simulink model "Project6"  (R2014a)
settings: Solver=ode45  StartTime=0.0  StopTime=310  RelTol=1e-3
undefined symbols (not defined in the file or in its folder): AXI4, Lite
libraries: xbsIndex_r4 x267
(part 1 of 2)
settings Model: Creator=Uday Kiran  LastModifiedBy=uk3
settings DebuggingCC: SolverPrmCheckMsg=none

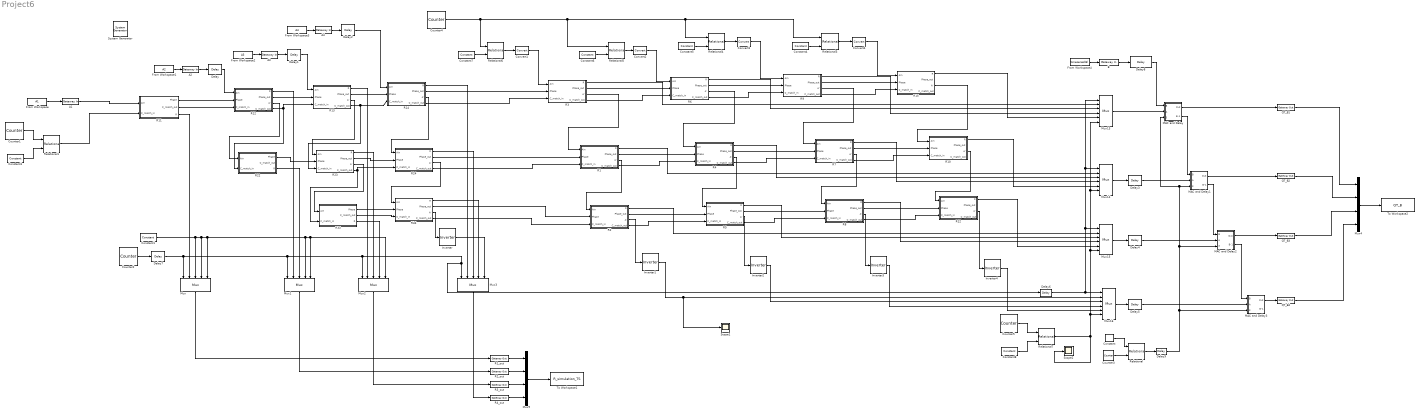
== system Project6 ==
  " System Generator" : xbsIndex_r4/ System Generator  Tag=genX  xilinxfamily=zynq  part=xc7z020  speed=-1  package=clg484  synthesis_tool=Vivado  clock_wrapper=Clock Enables  directory=./netlist  proj_type=Vivado  Synth_file=Vivado Synthesis Defaults  Impl_file=Vivado Implementation Defaults  testbench=off  simulink_period=1  sysclk_period=10  dcm_input_clock_period=10  incr_netlist=off  trim_vbits=Everywhere in SubSystem  dbl_ovrd=According to Block Masks  core_generation=According to Block Masks  run_coregen=off  deprecated_control=off  eval_field=0  block_type=sysgen
  A{1..4} (4 alike) : xbsIndex_r4/Gateway In  gui_display_data_type=Fixed-point  arith_type="Signed  (2's comp)"  n_bits=16  bin_pt=14  preci_type=Single  exp_width=8  frac_width=24  quantization="Round  (unbiased: +/- Inf)"  overflow=Saturate  period=1  UseAsADC=off  ADCChannel='1'  interface=AXI4-Lite  automatic_assignment=on  address_offset=hex2dec('00')  intf_description=''  timing_constraint=None  locs_specified=off  LOCs={}  io_standard={}  inherit_from_input=off  hdl_port=on  dbl_ovrd=off  block_type=gatewayin
      settings: block_version=VER_STRING_GOES_HERE
  B : xbsIndex_r4/Gateway In  gui_display_data_type=Fixed-point  arith_type="Signed  (2's comp)"  n_bits=16  bin_pt=14  preci_type=Single  exp_width=8  frac_width=24  quantization="Round  (unbiased: +/- Inf)"  overflow=Saturate  period=1  UseAsADC=off  ADCChannel='1'  interface=AXI4-Lite  automatic_assignment=on  address_offset=hex2dec('00')  intf_description=''  timing_constraint=None  locs_specified=off  LOCs={}  io_standard={}  inherit_from_input=off  hdl_port=on  dbl_ovrd=off  block_type=gatewayin
  Constant : xbsIndex_r4/Constant  const=8  gui_display_data_type=Fixed-point  arith_type=Signed (2's comp)  n_bits=16  bin_pt=0  preci_type=Single  exp_width=8  frac_width=24  explicit_period=on  period=1  equ=P=C  opselect=C  inp2=PCIN>>17  opr=+  inp1=P  carry=CIN  dbl_ovrd=off  block_type=constant
  Constant1 : xbsIndex_r4/Constant  const=0  gui_display_data_type=Fixed-point  arith_type=Signed (2's comp)  n_bits=16  bin_pt=14  preci_type=Single  exp_width=8  frac_width=24  explicit_period=off  period=1  equ=P=C  opselect=C  inp2=PCIN>>17  opr=+  inp1=P  carry=CIN  dbl_ovrd=off  block_type=constant
  Constant3 : xbsIndex_r4/Constant  const=0  gui_display_data_type=Fixed-point  arith_type=Signed (2's comp)  n_bits=8  bin_pt=0  preci_type=Single  exp_width=8  frac_width=24  explicit_period=off  period=1  equ=P=C  opselect=C  inp2=PCIN>>17  opr=+  inp1=P  carry=CIN  dbl_ovrd=off  block_type=constant
  Constant4 : xbsIndex_r4/Constant  const=7  gui_display_data_type=Fixed-point  arith_type=Signed (2's comp)  n_bits=10  bin_pt=0  preci_type=Single  exp_width=8  frac_width=24  explicit_period=off  period=1  equ=P=C  opselect=C  inp2=PCIN>>17  opr=+  inp1=P  carry=CIN  dbl_ovrd=off  block_type=constant
  Constant5 : xbsIndex_r4/Constant  const=54  gui_display_data_type=Fixed-point  arith_type=Signed (2's comp)  n_bits=10  bin_pt=0  preci_type=Single  exp_width=8  frac_width=24  explicit_period=off  period=1  equ=P=C  opselect=C  inp2=PCIN>>17  opr=+  inp1=P  carry=CIN  dbl_ovrd=off  block_type=constant
  Constant6 : xbsIndex_r4/Constant  const=101  gui_display_data_type=Fixed-point  arith_type=Signed (2's comp)  n_bits=10  bin_pt=0  preci_type=Single  exp_width=8  frac_width=24  explicit_period=off  period=1  equ=P=C  opselect=C  inp2=PCIN>>17  opr=+  inp1=P  carry=CIN  dbl_ovrd=off  block_type=constant
  Constant7 : xbsIndex_r4/Constant  const=148  gui_display_data_type=Fixed-point  arith_type=Signed (2's comp)  n_bits=10  bin_pt=0  preci_type=Single  exp_width=8  frac_width=24  explicit_period=off  period=1  equ=P=C  opselect=C  inp2=PCIN>>17  opr=+  inp1=P  carry=CIN  dbl_ovrd=off  block_type=constant
  Constant8 : xbsIndex_r4/Constant  const=296  gui_display_data_type=Fixed-point  arith_type=Signed (2's comp)  n_bits=10  bin_pt=0  preci_type=Single  exp_width=8  frac_width=24  explicit_period=off  period=1  equ=P=C  opselect=C  inp2=PCIN>>17  opr=+  inp1=P  carry=CIN  dbl_ovrd=off  block_type=constant
  Convert{1..4} (4 alike) : xbsIndex_r4/Convert  gui_display_data_type=Fixed-point  arith_type="Signed  (2's comp)"  n_bits=16  bin_pt=14  float_type=Single  exp_bits=8  fraction_bits=24  quantization=Truncate  overflow=Wrap  en=off  latency=0  pipeline=on  dbl_ovrd=off  block_type=convert
  Counter1 : xbsIndex_r4/Counter  cnt_type=Count Limited  cnt_to=47  operation=Up  start_count=0  cnt_by_val=1  arith_type="Signed  (2's comp)"  n_bits=8  bin_pt=0  load_pin=off  rst=off  en=off  explicit_period=on  period=1  use_behavioral_HDL=off  implementation=Fabric  dbl_ovrd=off  block_type=counter
  Counter2 : xbsIndex_r4/Counter  cnt_type=Count Limited  cnt_to=3  operation=Up  start_count=0  cnt_by_val=1  arith_type=Unsigned  n_bits=2  bin_pt=0  load_pin=off  rst=off  en=off  explicit_period=on  period=1  use_behavioral_HDL=off  implementation=Fabric  dbl_ovrd=off  block_type=counter
  Counter3 : xbsIndex_r4/Counter  cnt_type=Count Limited  cnt_to=8  operation=Up  start_count=1  cnt_by_val=1  arith_type=Unsigned  n_bits=5  bin_pt=0  load_pin=off  rst=off  en=off  explicit_period=on  period=1  use_behavioral_HDL=off  implementation=Fabric  dbl_ovrd=off  block_type=counter
  Counter4 : xbsIndex_r4/Counter  cnt_type=Count Limited  cnt_to=193  operation=Up  start_count=0  cnt_by_val=1  arith_type="Signed  (2's comp)"  n_bits=10  bin_pt=0  load_pin=off  rst=off  en=off  explicit_period=on  period=1  use_behavioral_HDL=off  implementation=Fabric  dbl_ovrd=off  block_type=counter
  Counter5 : xbsIndex_r4/Counter  cnt_type=Count Limited  cnt_to=300  operation=Up  start_count=1  cnt_by_val=1  arith_type="Signed  (2's comp)"  n_bits=10  bin_pt=0  load_pin=off  rst=off  en=off  explicit_period=on  period=1  use_behavioral_HDL=off  implementation=Fabric  dbl_ovrd=off  block_type=counter
  Delay : xbsIndex_r4/Delay  rst=off  infoeditControl=Selection of Reset will increase slice count due to use of real FFs and instead of SRLs  en=off  latency=1  reg_retiming=off  dbl_ovrd=off  block_type=delay
  Delay1 : xbsIndex_r4/Delay  rst=off  infoeditControl=Selection of Reset will increase slice count due to use of real FFs and instead of SRLs  en=off  latency=2  reg_retiming=off  dbl_ovrd=off  block_type=delay
  Delay2 : xbsIndex_r4/Delay  rst=off  infoeditControl=Selection of Reset will increase slice count due to use of real FFs and instead of SRLs  en=off  latency=3  reg_retiming=off  dbl_ovrd=off  block_type=delay
  Delay3 : xbsIndex_r4/Delay  rst=off  infoeditControl=Selection of Reset will increase slice count due to use of real FFs and instead of SRLs  en=off  latency=1  reg_retiming=off  dbl_ovrd=off  block_type=delay
  Delay4 : xbsIndex_r4/Delay  rst=off  infoeditControl=Selection of Reset will increase slice count due to use of real FFs and instead of SRLs  en=off  latency=2  reg_retiming=off  dbl_ovrd=off  block_type=delay
  Delay5 : xbsIndex_r4/Delay  rst=off  infoeditControl=Selection of Reset will increase slice count due to use of real FFs and instead of SRLs  en=off  latency=3  reg_retiming=off  dbl_ovrd=off  block_type=delay
  Delay6 : xbsIndex_r4/Delay  rst=off  infoeditControl=Selection of Reset will increase slice count due to use of real FFs and instead of SRLs  en=off  latency=3  reg_retiming=off  dbl_ovrd=off  block_type=delay
  Delay7 : xbsIndex_r4/Delay  rst=off  infoeditControl=Selection of Reset will increase slice count due to use of real FFs and instead of SRLs  en=off  latency=1  reg_retiming=off  dbl_ovrd=off  block_type=delay
  Delay8 : xbsIndex_r4/Delay  rst=off  infoeditControl=Selection of Reset will increase slice count due to use of real FFs and instead of SRLs  en=off  latency=297  reg_retiming=off  dbl_ovrd=off  block_type=delay
  Delay9 : xbsIndex_r4/Delay  rst=off  infoeditControl=Selection of Reset will increase slice count due to use of real FFs and instead of SRLs  en=off  latency=4  reg_retiming=off  dbl_ovrd=off  block_type=delay
  From Workspace : FromWorkspace  VariableName=A1  SampleTime=0  OutputAfterFinalValue=Setting to zero
  From Workspace1 : FromWorkspace  VariableName=A2  SampleTime=0  OutputAfterFinalValue=Setting to zero
  From Workspace2 : FromWorkspace  VariableName=A3  SampleTime=0  OutputAfterFinalValue=Setting to zero
  From Workspace3 : FromWorkspace  VariableName=A4  SampleTime=0  OutputAfterFinalValue=Setting to zero
  From Workspace4 : FromWorkspace  VariableName=timeseries(B)  SampleTime=0  OutputAfterFinalValue=Setting to zero
  Inverter{,1..4} (5 alike) : xbsIndex_r4/Inverter  en=off  latency=0  dbl_ovrd=off  block_type=inv
  MAC and Delay : Subsystem
  MAC and Delay1 : Subsystem
  MAC and Delay2 : Subsystem
  MAC and Delay3 : Subsystem
  Mux{,1..3} (4 alike) : xbsIndex_r4/Mux  inputs=4  en=off  latency=0  precision=Full  arith_type=Unsigned  n_bits=16  bin_pt=14  quantization=Truncate  overflow=Wrap  dbl_ovrd=off  block_type=mux
  Mux{13..16} (4 alike) : xbsIndex_r4/Mux  inputs=4  en=on  latency=1  precision=User Defined  arith_type="Signed  (2's comp)"  n_bits=16  bin_pt=14  quantization=Truncate  overflow=Wrap  dbl_ovrd=off  block_type=mux
  Mux4 : Mux
  Mux9 : Mux
  QT_B{1..4} (4 alike) : xbsIndex_r4/Gateway Out  inherit_from_input=off  hdl_port=on  rows=1  columns=1  UseAsDAC=off  DACChannel='1'  interface=AXI4-Lite  automatic_assignment=on  address_offset=hex2dec('00')  intf_description=''  timing_constraint=None  locs_specified=off  LOCs={}  io_standard={}  block_type=gatewayout
  R1 : Subsystem
  R10 : Subsystem
  R11 : Subsystem
  R12 : Subsystem
  "R12 " : Subsystem
  R13 : Subsystem
  R14 : Subsystem
  R15 : Subsystem
  R1_out : xbsIndex_r4/Gateway Out  inherit_from_input=off  hdl_port=on  rows=1  columns=1  UseAsDAC=off  DACChannel='1'  interface=AXI4-Lite  automatic_assignment=on  address_offset=hex2dec('00')  intf_description=''  timing_constraint=None  locs_specified=off  LOCs={}  io_standard={}  block_type=gatewayout
  R2 : Subsystem
  R22 : Subsystem
  R23 : Subsystem
  R24 : Subsystem
  R2_out : xbsIndex_r4/Gateway Out  inherit_from_input=off  hdl_port=on  rows=1  columns=1  UseAsDAC=off  DACChannel='1'  interface=AXI4-Lite  automatic_assignment=on  address_offset=hex2dec('00')  intf_description=''  timing_constraint=None  locs_specified=off  LOCs={}  io_standard={}  block_type=gatewayout
  R3 : Subsystem
  R33 : Subsystem
  R34 : Subsystem
  R3_out : xbsIndex_r4/Gateway Out  inherit_from_input=off  hdl_port=on  rows=1  columns=1  UseAsDAC=off  DACChannel='1'  interface=AXI4-Lite  automatic_assignment=on  address_offset=hex2dec('00')  intf_description=''  timing_constraint=None  locs_specified=off  LOCs={}  io_standard={}  block_type=gatewayout
  R4 : Subsystem
  R4_out : xbsIndex_r4/Gateway Out  inherit_from_input=off  hdl_port=on  rows=1  columns=1  UseAsDAC=off  DACChannel='1'  interface=AXI4-Lite  automatic_assignment=on  address_offset=hex2dec('00')  intf_description=''  timing_constraint=None  locs_specified=off  LOCs={}  io_standard={}  block_type=gatewayout
  R5 : Subsystem
  R6 : Subsystem
  R7 : Subsystem
  R8 : Subsystem
  R9 : Subsystem
  Relational{,1,3..6} (6 alike) : xbsIndex_r4/Relational  mode=a=b  op_type=Bool  en=off  latency=0  dbl_ovrd=off  block_type=relational
  Relational7 : xbsIndex_r4/Relational  mode=a>b  op_type=Bool  en=off  latency=0  dbl_ovrd=off  block_type=relational
  Scope1 : Scope
  Scope2 : Scope
  To Workspace1 : ToWorkspace  VariableName=R_simulation_TS  SaveFormat=Timeseries  SampleTime=-1
      settings: MaxDataPoints=8
  To Workspace2 : ToWorkspace  VariableName=QT_B  SaveFormat=Timeseries  SampleTime=-1
  wires:
  From Workspace/1 -> A1/1
  From Workspace1/1 -> A2/1
  A1/1 -> R11/1(Ain)
  A2/1 -> Delay/1
  R11/1(Phase) -> "R12 "/2(Phase)
  R11/2(C_match_out) -> "R12 "/3(C_match_in)
  Counter1/1 -> Relational1/1
  Constant3/1 -> Relational1/2
  Relational1/1 -> R11/2("C_match_in ")
  "R12 "/3(A') -> R22/1(Ain)
  "R12 "/4(C_match_out) -> R22/2("C_match_in "), R13/3(C_match_in)
  Delay/1 -> "R12 "/1(Ain)
  "R12 "/2(Phase_out) -> R13/2(Phase)
  R13/2(Phase_out) -> R14/2(Phase)
  R13/3(A') -> R23/1(Ain)
  R23/2(Phase_out) -> R24/2(Phase)
  R14/3(A') -> R24/1(Ain)
  R23/3(A') -> R33/1(Ain)
  R23/4(C_match_out) -> R33/2("C_match_in "), R24/3(C_match_in)
  R33/1(Phase) -> R34/2(Phase)
  R24/3(A') -> R34/1(Ain)
  From Workspace2/1 -> A3/1
  A3/1 -> Delay1/1
  Delay1/1 -> R13/1(Ain)
  From Workspace3/1 -> A4/1
  A4/1 -> Delay2/1
  Delay2/1 -> R14/1(Ain)
  "R12 "/1(R) -> Mux1/2
  R22/3(R) -> Mux1/3
  R13/1(R) -> Mux2/2
  R23/1(R) -> Mux2/3
  R33/3(R) -> Mux2/4
  R14/1(R) -> Mux3/2
  R24/1(R) -> Mux3/3
  R34/1(R) -> Mux3/4
  R34/3(A') -> Inverter/1
  R33/2(C_match_out) -> R34/3(C_match_in)
  R13/4(C_match_out) -> R14/3(C_match_in), R23/3(C_match_in)
  R22/1(Phase) -> R23/2(Phase)
  R3/3(A') -> R1/1(Ain)
  R1/3(A') -> R2/1(Ain)
  R6/3(A') -> R4/1(Ain)
  R4/3(A') -> R5/1(Ain)
  R9/3(A') -> R7/1(Ain)
  R7/3(A') -> R8/1(Ain)
  R15/3(A') -> R10/1(Ain)
  R10/3(A') -> R12/1(Ain)
  R14/2(Phase_out) -> R3/2(Phase)
  R3/2(Phase_out) -> R6/2(Phase)
  R6/2(Phase_out) -> R9/2(Phase)
  R9/2(Phase_out) -> R15/2(Phase)
  R24/2(Phase_out) -> R1/2(Phase)
  R1/2(Phase_out) -> R4/2(Phase)
  R4/2(Phase_out) -> R7/2(Phase)
  R7/2(Phase_out) -> R10/2(Phase)
  R34/2(Phase_out) -> R2/2(Phase)
  R2/2(Phase_out) -> R5/2(Phase)
  R5/2(Phase_out) -> R8/2(Phase)
  R8/2(Phase_out) -> R12/2(Phase)
  R14/4(C_match_out) -> R3/3(C_match_in)
  R24/4(C_match_out) -> R1/3(C_match_in)
  R34/4(C_match_out) -> R2/3(C_match_in)
  R3/4(C_match_out) -> R6/3(C_match_in)
  R6/4(C_match_out) -> R9/3(C_match_in)
  R9/4(C_match_out) -> R15/3(C_match_in)
  R1/4(C_match_out) -> R4/3(C_match_in)
  R4/4(C_match_out) -> R7/3(C_match_in)
  R7/4(C_match_out) -> R10/3(C_match_in)
  R2/4(C_match_out) -> R5/3(C_match_in)
  R5/4(C_match_out) -> R8/3(C_match_in)
  R8/4(C_match_out) -> R12/3(C_match_in)
  R3/1(R) -> Mux13/2
  R1/1(R) -> Mux14/2
  R2/1(R) -> Mux15/2
  R2/3(A') -> Inverter1/1
  R6/1(R) -> Mux13/3
  R4/1(R) -> Mux14/3
  R5/1(R) -> Mux15/3
  R5/3(A') -> Inverter2/1
  R9/1(R) -> Mux13/4
  R7/1(R) -> Mux14/4
  R8/1(R) -> Mux15/4
  R8/3(A') -> Inverter3/1
  R10/1(R) -> Mux14/5
  R12/1(R) -> Mux15/5
  R12/3(A') -> Inverter4/1
  R11/3(R) -> Mux/2
  Inverter/1 -> Mux3/5
  Counter2/1 -> Delay7/1
  Mux/1 -> R1_out/1
  Mux1/1 -> R2_out/1
  Mux2/1 -> R3_out/1
  Mux3/1 -> R4_out/1
  R1_out/1 -> Mux9/1
  R2_out/1 -> Mux9/2
  R3_out/1 -> Mux9/3
  R4_out/1 -> Mux9/4
  Mux9/1 -> To Workspace1/1
  Constant1/1 -> Mux1/5, Mux2/5, Mux1/4, Mux/5, Mux/4, Mux/3
  Constant4/1 -> Relational3/2
  Constant5/1 -> Relational4/2
  Constant6/1 -> Relational5/2
  Counter4/1 -> Relational3/1, Relational4/1, Relational5/1, Relational6/1
  Constant7/1 -> Relational6/2
  Relational6/1 -> Convert1/1
  Relational5/1 -> Convert2/1
  Relational4/1 -> Convert3/1
  Relational3/1 -> Convert4/1
  Convert1/1 -> R3/1(Ain)
  Convert2/1 -> R6/1(Ain)
  Convert3/1 -> R9/1(Ain)
  Convert4/1 -> R15/1(Ain)
  Mux14/1 -> Delay3/1
  Mux15/1 -> Delay4/1
  From Workspace4/1 -> B/1
  B/1 -> Delay8/1
  Mux13/1 -> MAC and Delay/2(A)
  MAC and Delay/1("Out ") -> QT_B1/1
  MAC and Delay/2(B-1) -> MAC and Delay1/1(B)
  Delay3/1 -> MAC and Delay1/2(A)
  Delay4/1 -> MAC and Delay2/2(A)
  MAC and Delay1/1("Out ") -> QT_B2/1
  MAC and Delay1/2(B-1) -> MAC and Delay2/1(B)
  MAC and Delay2/1("Out ") -> QT_B3/1
  MAC and Delay2/2(B-1) -> MAC and Delay3/1(B)
  Delay5/1 -> MAC and Delay3/2(A)
  MAC and Delay3/1("Out ") -> QT_B4/1
  R15/1(R) -> Mux13/5
  Inverter1/1 -> Scope1/1, Mux16/2
  Inverter2/1 -> Mux16/3
  Inverter3/1 -> Mux16/4
  Inverter4/1 -> Mux16/5
  Delay8/1 -> MAC and Delay/1(B)
  QT_B1/1 -> Mux4/1
  QT_B2/1 -> Mux4/2
  QT_B3/1 -> Mux4/3
  QT_B4/1 -> Mux4/4
  Mux4/1 -> To Workspace2/1
  Delay7/1 -> Mux/1, Mux2/1, Mux3/1, Delay6/1, Mux1/1
  Counter5/1 -> Relational7/1
  Constant8/1 -> Relational7/2
  Relational7/1 -> Scope2/1, Mux15/6, Mux14/6, Mux13/6, Mux16/6
  Mux16/1 -> Delay5/1
  Delay6/1 -> Mux15/1, Mux14/1, Mux13/1, Mux16/1
  Constant/1 -> Relational/1
  Counter3/1 -> Relational/2
  Relational/1 -> Delay9/1
  Delay9/1 -> MAC and Delay3/3(AccRst), MAC and Delay/3(AccRst), MAC and Delay1/3(AccRst), MAC and Delay2/3(AccRst)

== system Project6/MAC and Delay ==
  B : Inport
  A : Inport  Port=2
  AccRst : Inport  Port=3
  Accumulator : xbsIndex_r4/Accumulator  operation=Add  n_bits=16  overflow=Wrap  scale=1  rst=on  hasbypass=off  infoeditControl=reset for floating point data type must be asserted for a minimum of 2 cycles  en=off  latency=1  msb_inp=100  msb=100  lsb=-100  use_behavioral_HDL=on  implementation=Fabric  dbl_ovrd=off  block_type=accum
  Delay3 : xbsIndex_r4/Delay  rst=off  infoeditControl=Selection of Reset will increase slice count due to use of real FFs and instead of SRLs  en=off  latency=1  reg_retiming=off  dbl_ovrd=off  block_type=delay
  Mult : xbsIndex_r4/Mult  precision=User Defined  arith_type="Signed  (2's comp)"  n_bits=16  bin_pt=14  quantization=Truncate  overflow=Wrap  en=off  latency=3  use_behavioral_HDL=off  opt=Speed  use_embedded=on  optimum_pipeline=off  pipeline=on  dbl_ovrd=off  use_rpm=on  placement_style=Triangular  block_type=mult
  "Out " : Outport
  B-1 : Outport  Port=2
  wires:
  AccRst/1 -> Accumulator/2
  A/1 -> Mult/1
  Accumulator/1 -> "Out "/1
  Delay3/1 -> B-1/1
  B/1 -> Delay3/1, Mult/2
  Mult/1 -> Accumulator/1

== system Project6/MAC and Delay1 ==
  B : Inport
  A : Inport  Port=2
  AccRst : Inport  Port=3
  Accumulator : xbsIndex_r4/Accumulator  operation=Add  n_bits=16  overflow=Wrap  scale=1  rst=on  hasbypass=off  infoeditControl=reset for floating point data type must be asserted for a minimum of 2 cycles  en=off  latency=1  msb_inp=100  msb=100  lsb=-100  use_behavioral_HDL=on  implementation=Fabric  dbl_ovrd=off  block_type=accum
  Delay3 : xbsIndex_r4/Delay  rst=off  infoeditControl=Selection of Reset will increase slice count due to use of real FFs and instead of SRLs  en=off  latency=1  reg_retiming=off  dbl_ovrd=off  block_type=delay
  Mult : xbsIndex_r4/Mult  precision=User Defined  arith_type="Signed  (2's comp)"  n_bits=16  bin_pt=14  quantization=Truncate  overflow=Wrap  en=off  latency=3  use_behavioral_HDL=off  opt=Speed  use_embedded=on  optimum_pipeline=off  pipeline=on  dbl_ovrd=off  use_rpm=on  placement_style=Triangular  block_type=mult
  "Out " : Outport
  B-1 : Outport  Port=2
  wires:
  AccRst/1 -> Accumulator/2
  A/1 -> Mult/1
  Accumulator/1 -> "Out "/1
  Delay3/1 -> B-1/1
  B/1 -> Delay3/1, Mult/2
  Mult/1 -> Accumulator/1

== system Project6/MAC and Delay2 ==
  B : Inport
  A : Inport  Port=2
  AccRst : Inport  Port=3
  Accumulator : xbsIndex_r4/Accumulator  operation=Add  n_bits=16  overflow=Wrap  scale=1  rst=on  hasbypass=off  infoeditControl=reset for floating point data type must be asserted for a minimum of 2 cycles  en=off  latency=1  msb_inp=100  msb=100  lsb=-100  use_behavioral_HDL=on  implementation=Fabric  dbl_ovrd=off  block_type=accum
  Delay3 : xbsIndex_r4/Delay  rst=off  infoeditControl=Selection of Reset will increase slice count due to use of real FFs and instead of SRLs  en=off  latency=1  reg_retiming=off  dbl_ovrd=off  block_type=delay
  Mult : xbsIndex_r4/Mult  precision=User Defined  arith_type="Signed  (2's comp)"  n_bits=16  bin_pt=14  quantization=Truncate  overflow=Wrap  en=off  latency=3  use_behavioral_HDL=off  opt=Speed  use_embedded=on  optimum_pipeline=off  pipeline=on  dbl_ovrd=off  use_rpm=on  placement_style=Triangular  block_type=mult
  "Out " : Outport
  B-1 : Outport  Port=2
  wires:
  AccRst/1 -> Accumulator/2
  A/1 -> Mult/1
  Accumulator/1 -> "Out "/1
  Delay3/1 -> B-1/1
  B/1 -> Delay3/1, Mult/2
  Mult/1 -> Accumulator/1

== system Project6/MAC and Delay3 ==
  B : Inport
  A : Inport  Port=2
  AccRst : Inport  Port=3
  Accumulator : xbsIndex_r4/Accumulator  operation=Add  n_bits=16  overflow=Wrap  scale=1  rst=on  hasbypass=off  infoeditControl=reset for floating point data type must be asserted for a minimum of 2 cycles  en=off  latency=1  msb_inp=100  msb=100  lsb=-100  use_behavioral_HDL=on  implementation=Fabric  dbl_ovrd=off  block_type=accum
  Delay3 : xbsIndex_r4/Delay  rst=off  infoeditControl=Selection of Reset will increase slice count due to use of real FFs and instead of SRLs  en=off  latency=1  reg_retiming=off  dbl_ovrd=off  block_type=delay
  Mult : xbsIndex_r4/Mult  precision=User Defined  arith_type="Signed  (2's comp)"  n_bits=16  bin_pt=14  quantization=Truncate  overflow=Wrap  en=off  latency=3  use_behavioral_HDL=off  opt=Speed  use_embedded=on  optimum_pipeline=off  pipeline=on  dbl_ovrd=off  use_rpm=on  placement_style=Triangular  block_type=mult
  "Out " : Outport
  B-1 : Outport  Port=2
  wires:
  AccRst/1 -> Accumulator/2
  A/1 -> Mult/1
  Accumulator/1 -> "Out "/1
  Delay3/1 -> B-1/1
  B/1 -> Delay3/1, Mult/2
  Mult/1 -> Accumulator/1

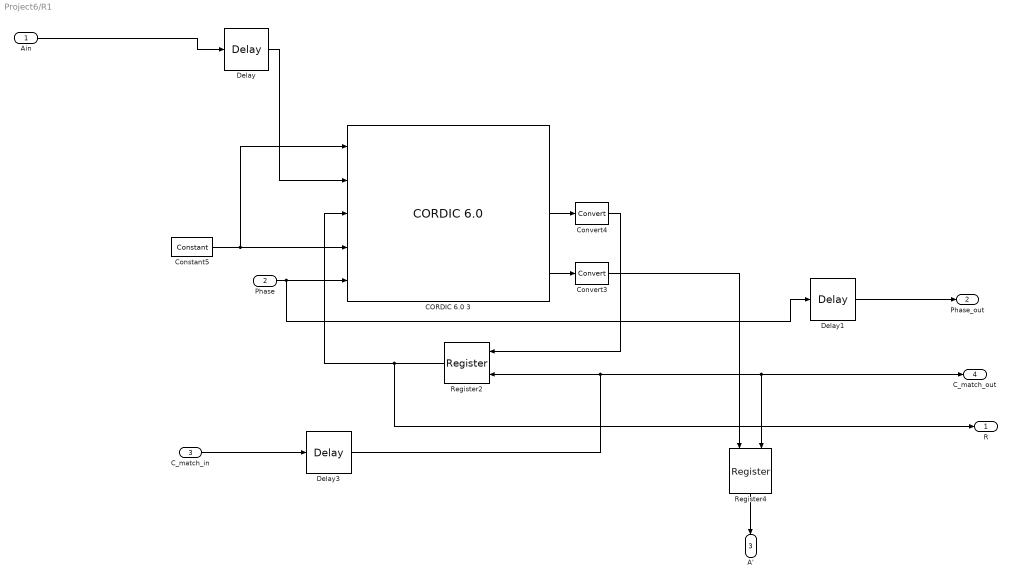
== system Project6/R1 ==
  Ain : Inport
  Phase : Inport  Port=2
  C_match_in : Inport  Port=3
  CORDIC 6.0 3 : xbsIndex_r4/CORDIC 6.0   functional_selection=Rotate  architectural_configuration=Parallel  pipelining_mode=Maximum  data_format=SignedFraction  phase_format=Radians  input_width=16  output_width=16  round_mode=Truncate  iterations=16  precision=16  compensation_scaling=LUT_based  coarse_rotation=on  aclken=off  aresetn=off  out_tready=off  cartesian_has_tuser=off  cartesian_has_tlast=off  cartesian_tuser_width=1  phase_has_tuser=off  phase_has_tlast=off  phase_tuser_width=1  out_tlast_behv=Null  flow_control=NonBlocking  optimize_goal=Performance  trim_axipin_name=on  ip_name=CORDIC  ip_version=6.0  dsptool_ready=true  ipcore_usecache=true  ipcore_useipmodelcache=true  wrapper_available=true  port_translation_map={ 'aclken' => 'en', 'aresetn' => 'rst' }  block_type=cordic_v6_0
      settings: infoedit=CORDIC 6.0
  Constant5 : xbsIndex_r4/Constant  const=1  gui_display_data_type=Boolean  arith_type=Boolean  n_bits=16  bin_pt=14  preci_type=Single  exp_width=8  frac_width=24  explicit_period=on  period=1  equ=P=C  opselect=C  inp2=PCIN>>17  opr=+  inp1=P  carry=CIN  dbl_ovrd=off  block_type=constant
  Convert3 : xbsIndex_r4/Convert  gui_display_data_type=Fixed-point  arith_type="Signed  (2's comp)"  n_bits=16  bin_pt=14  float_type=Single  exp_bits=8  fraction_bits=24  quantization=Truncate  overflow=Wrap  en=off  latency=0  pipeline=on  dbl_ovrd=off  block_type=convert
  Convert4 : xbsIndex_r4/Convert  gui_display_data_type=Fixed-point  arith_type="Signed  (2's comp)"  n_bits=16  bin_pt=14  float_type=Single  exp_bits=8  fraction_bits=24  quantization=Truncate  overflow=Wrap  en=off  latency=0  pipeline=on  dbl_ovrd=off  block_type=convert
  Delay : xbsIndex_r4/Delay  rst=off  infoeditControl=Selection of Reset will increase slice count due to use of real FFs and instead of SRLs  en=off  latency=22  reg_retiming=off  dbl_ovrd=off  block_type=delay
  Delay1 : xbsIndex_r4/Delay  rst=off  infoeditControl=Selection of Reset will increase slice count due to use of real FFs and instead of SRLs  en=off  latency=1  reg_retiming=off  dbl_ovrd=off  block_type=delay
  Delay3 : xbsIndex_r4/Delay  rst=off  infoeditControl=Selection of Reset will increase slice count due to use of real FFs and instead of SRLs  en=off  latency=1  reg_retiming=off  dbl_ovrd=off  block_type=delay
  Register2 : xbsIndex_r4/Register  init=0  rst=off  en=on  dbl_ovrd=off  block_type=register
  Register4 : xbsIndex_r4/Register  init=0  rst=off  en=on  dbl_ovrd=off  block_type=register
  R : Outport
  Phase_out : Outport  Port=2
  A' : Outport  Port=3
  C_match_out : Outport  Port=4
  wires:
  Ain/1 -> Delay/1
  Delay/1 -> CORDIC 6.0 3/2
  Convert4/1 -> Register2/1
  CORDIC 6.0 3/2 -> Convert4/1
  Register2/1 -> R/1, CORDIC 6.0 3/3
  CORDIC 6.0 3/3 -> Convert3/1
  Constant5/1 -> CORDIC 6.0 3/1, CORDIC 6.0 3/4
  Register4/1 -> A'/1
  Convert3/1 -> Register4/1
  Phase/1 -> Delay1/1, CORDIC 6.0 3/5
  Delay3/1 -> Register2/2, C_match_out/1, Register4/2
  C_match_in/1 -> Delay3/1
  Delay1/1 -> Phase_out/1

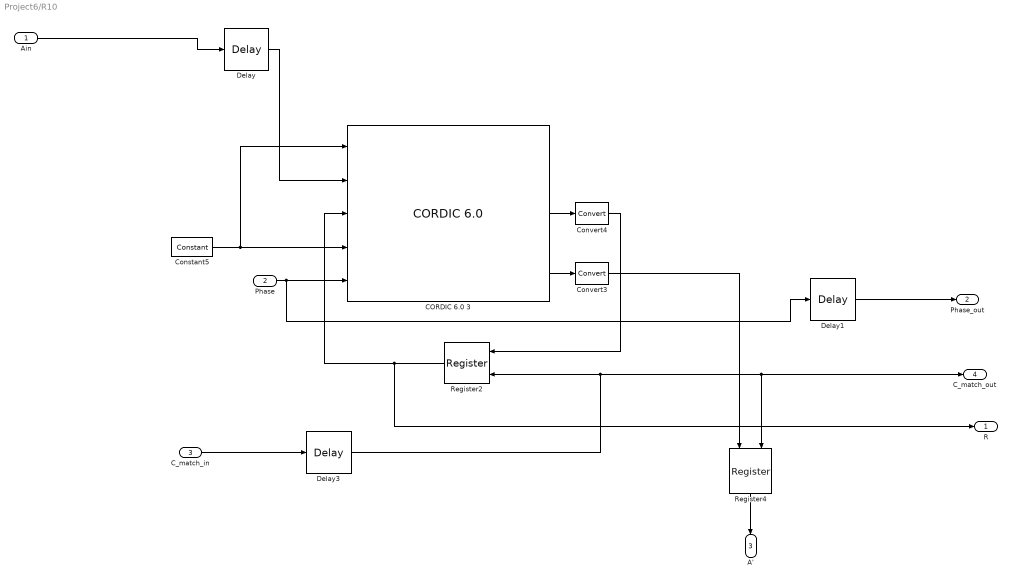
== system Project6/R10 ==
  Ain : Inport
  Phase : Inport  Port=2
  C_match_in : Inport  Port=3
  CORDIC 6.0 3 : xbsIndex_r4/CORDIC 6.0   functional_selection=Rotate  architectural_configuration=Parallel  pipelining_mode=Maximum  data_format=SignedFraction  phase_format=Radians  input_width=16  output_width=16  round_mode=Truncate  iterations=16  precision=16  compensation_scaling=LUT_based  coarse_rotation=on  aclken=off  aresetn=off  out_tready=off  cartesian_has_tuser=off  cartesian_has_tlast=off  cartesian_tuser_width=1  phase_has_tuser=off  phase_has_tlast=off  phase_tuser_width=1  out_tlast_behv=Null  flow_control=NonBlocking  optimize_goal=Performance  trim_axipin_name=on  ip_name=CORDIC  ip_version=6.0  dsptool_ready=true  ipcore_usecache=true  ipcore_useipmodelcache=true  wrapper_available=true  port_translation_map={ 'aclken' => 'en', 'aresetn' => 'rst' }  block_type=cordic_v6_0
      settings: infoedit=CORDIC 6.0
  Constant5 : xbsIndex_r4/Constant  const=1  gui_display_data_type=Boolean  arith_type=Boolean  n_bits=16  bin_pt=14  preci_type=Single  exp_width=8  frac_width=24  explicit_period=on  period=1  equ=P=C  opselect=C  inp2=PCIN>>17  opr=+  inp1=P  carry=CIN  dbl_ovrd=off  block_type=constant
  Convert3 : xbsIndex_r4/Convert  gui_display_data_type=Fixed-point  arith_type="Signed  (2's comp)"  n_bits=16  bin_pt=14  float_type=Single  exp_bits=8  fraction_bits=24  quantization=Truncate  overflow=Wrap  en=off  latency=0  pipeline=on  dbl_ovrd=off  block_type=convert
  Convert4 : xbsIndex_r4/Convert  gui_display_data_type=Fixed-point  arith_type="Signed  (2's comp)"  n_bits=16  bin_pt=14  float_type=Single  exp_bits=8  fraction_bits=24  quantization=Truncate  overflow=Wrap  en=off  latency=0  pipeline=on  dbl_ovrd=off  block_type=convert
  Delay : xbsIndex_r4/Delay  rst=off  infoeditControl=Selection of Reset will increase slice count due to use of real FFs and instead of SRLs  en=off  latency=22  reg_retiming=off  dbl_ovrd=off  block_type=delay
  Delay1 : xbsIndex_r4/Delay  rst=off  infoeditControl=Selection of Reset will increase slice count due to use of real FFs and instead of SRLs  en=off  latency=1  reg_retiming=off  dbl_ovrd=off  block_type=delay
  Delay3 : xbsIndex_r4/Delay  rst=off  infoeditControl=Selection of Reset will increase slice count due to use of real FFs and instead of SRLs  en=off  latency=1  reg_retiming=off  dbl_ovrd=off  block_type=delay
  Register2 : xbsIndex_r4/Register  init=0  rst=off  en=on  dbl_ovrd=off  block_type=register
  Register4 : xbsIndex_r4/Register  init=0  rst=off  en=on  dbl_ovrd=off  block_type=register
  R : Outport
  Phase_out : Outport  Port=2
  A' : Outport  Port=3
  C_match_out : Outport  Port=4
  wires:
  Ain/1 -> Delay/1
  Delay/1 -> CORDIC 6.0 3/2
  Convert4/1 -> Register2/1
  CORDIC 6.0 3/2 -> Convert4/1
  Register2/1 -> R/1, CORDIC 6.0 3/3
  CORDIC 6.0 3/3 -> Convert3/1
  Constant5/1 -> CORDIC 6.0 3/1, CORDIC 6.0 3/4
  Register4/1 -> A'/1
  Convert3/1 -> Register4/1
  Phase/1 -> Delay1/1, CORDIC 6.0 3/5
  Delay3/1 -> Register2/2, C_match_out/1, Register4/2
  C_match_in/1 -> Delay3/1
  Delay1/1 -> Phase_out/1

== system Project6/R11 ==
  Ain : Inport
  "C_match_in " : Inport  Port=2
  CORDIC 6.0 1 : xbsIndex_r4/CORDIC 6.0   functional_selection=Rotate  architectural_configuration=Parallel  pipelining_mode=Maximum  data_format=SignedFraction  phase_format=Radians  input_width=16  output_width=16  round_mode=Truncate  iterations=16  precision=16  compensation_scaling=LUT_based  coarse_rotation=on  aclken=off  aresetn=off  out_tready=off  cartesian_has_tuser=off  cartesian_has_tlast=off  cartesian_tuser_width=1  phase_has_tuser=off  phase_has_tlast=off  phase_tuser_width=1  out_tlast_behv=Null  flow_control=NonBlocking  optimize_goal=Performance  trim_axipin_name=on  ip_name=CORDIC  ip_version=6.0  dsptool_ready=true  ipcore_usecache=true  ipcore_useipmodelcache=true  wrapper_available=true  port_translation_map={ 'aclken' => 'en', 'aresetn' => 'rst' }  block_type=cordic_v6_0
      settings: infoedit=CORDIC 6.0
  CORDIC 6.0 2 : xbsIndex_r4/CORDIC 6.0   functional_selection=Arc_Tan  architectural_configuration=Parallel  pipelining_mode=Maximum  data_format=SignedFraction  phase_format=Radians  input_width=16  output_width=16  round_mode=Truncate  iterations=16  precision=16  compensation_scaling=No_Scale_Compensation  coarse_rotation=on  aclken=off  aresetn=off  out_tready=off  cartesian_has_tuser=off  cartesian_has_tlast=off  cartesian_tuser_width=1  phase_has_tuser=off  phase_has_tlast=off  phase_tuser_width=1  out_tlast_behv=Null  flow_control=NonBlocking  optimize_goal=Performance  trim_axipin_name=on  ip_name=CORDIC  ip_version=6.0  dsptool_ready=true  ipcore_usecache=true  ipcore_useipmodelcache=true  wrapper_available=true  port_translation_map={ 'aclken' => 'en', 'aresetn' => 'rst' }  block_type=cordic_v6_0
      settings: infoedit=CORDIC 6.0
  Constant1 : xbsIndex_r4/Constant  const=1  gui_display_data_type=Boolean  arith_type=Boolean  n_bits=16  bin_pt=14  preci_type=Single  exp_width=8  frac_width=24  explicit_period=on  period=1  equ=P=C  opselect=C  inp2=PCIN>>17  opr=+  inp1=P  carry=CIN  dbl_ovrd=off  block_type=constant
  Constant2 : xbsIndex_r4/Constant  const=1  gui_display_data_type=Boolean  arith_type=Boolean  n_bits=16  bin_pt=14  preci_type=Single  exp_width=8  frac_width=24  explicit_period=on  period=1  equ=P=C  opselect=C  inp2=PCIN>>17  opr=+  inp1=P  carry=CIN  dbl_ovrd=off  block_type=constant
  Convert1 : xbsIndex_r4/Convert  gui_display_data_type=Fixed-point  arith_type="Signed  (2's comp)"  n_bits=16  bin_pt=14  float_type=Single  exp_bits=8  fraction_bits=24  quantization=Truncate  overflow=Wrap  en=off  latency=0  pipeline=on  dbl_ovrd=off  block_type=convert
  Convert2 : xbsIndex_r4/Convert  gui_display_data_type=Fixed-point  arith_type="Signed  (2's comp)"  n_bits=16  bin_pt=14  float_type=Single  exp_bits=8  fraction_bits=24  quantization=Truncate  overflow=Wrap  en=off  latency=0  pipeline=on  dbl_ovrd=off  block_type=convert
  Delay1 : xbsIndex_r4/Delay  rst=off  infoeditControl=Selection of Reset will increase slice count due to use of real FFs and instead of SRLs  en=off  latency=1  reg_retiming=off  dbl_ovrd=off  block_type=delay
  Register : xbsIndex_r4/Register  init=0  rst=off  en=on  dbl_ovrd=off  block_type=register
  Register1 : xbsIndex_r4/Register  init=0  rst=off  en=on  dbl_ovrd=off  block_type=register
  Phase : Outport
  C_match_out : Outport  Port=2
  R : Outport  Port=3
  wires:
  Constant1/1 -> CORDIC 6.0 1/1, CORDIC 6.0 1/4
  Constant2/1 -> CORDIC 6.0 2/1
  Delay1/1 -> Phase/1
  CORDIC 6.0 1/2 -> Convert2/1
  CORDIC 6.0 2/2 -> Delay1/1, CORDIC 6.0 1/5
  Register1/1 -> CORDIC 6.0 2/3, CORDIC 6.0 1/2
  Convert1/1 -> CORDIC 6.0 2/2
  Ain/1 -> Register1/1
  Register/1 -> R/1, Convert1/1, CORDIC 6.0 1/3
  Convert2/1 -> Register/1
  "C_match_in "/1 -> Register1/2, Register/2, C_match_out/1

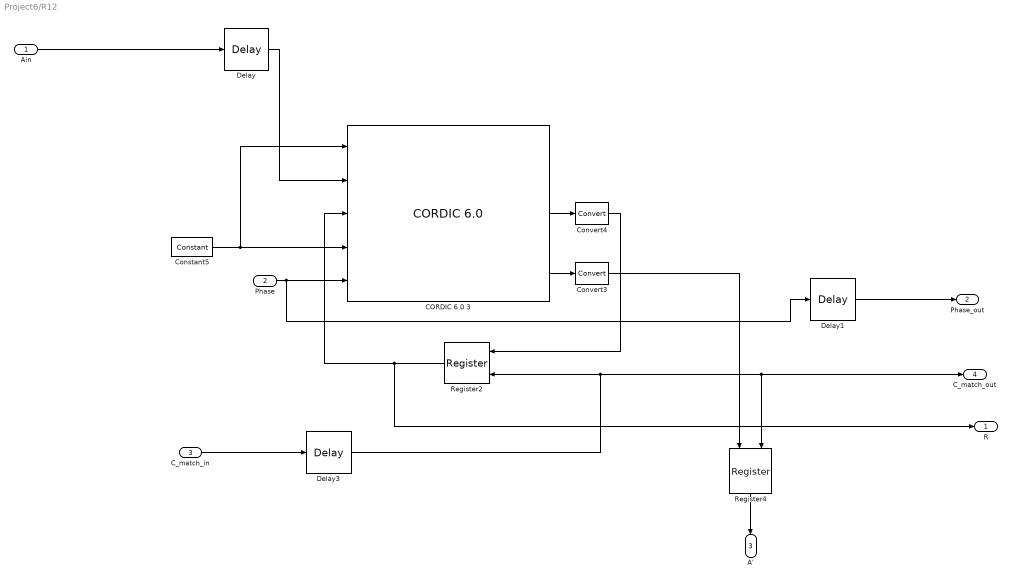
== system Project6/R12 ==
  Ain : Inport
  Phase : Inport  Port=2
  C_match_in : Inport  Port=3
  CORDIC 6.0 3 : xbsIndex_r4/CORDIC 6.0   functional_selection=Rotate  architectural_configuration=Parallel  pipelining_mode=Maximum  data_format=SignedFraction  phase_format=Radians  input_width=16  output_width=16  round_mode=Truncate  iterations=16  precision=16  compensation_scaling=LUT_based  coarse_rotation=on  aclken=off  aresetn=off  out_tready=off  cartesian_has_tuser=off  cartesian_has_tlast=off  cartesian_tuser_width=1  phase_has_tuser=off  phase_has_tlast=off  phase_tuser_width=1  out_tlast_behv=Null  flow_control=NonBlocking  optimize_goal=Performance  trim_axipin_name=on  ip_name=CORDIC  ip_version=6.0  dsptool_ready=true  ipcore_usecache=true  ipcore_useipmodelcache=true  wrapper_available=true  port_translation_map={ 'aclken' => 'en', 'aresetn' => 'rst' }  block_type=cordic_v6_0
      settings: infoedit=CORDIC 6.0
  Constant5 : xbsIndex_r4/Constant  const=1  gui_display_data_type=Boolean  arith_type=Boolean  n_bits=16  bin_pt=14  preci_type=Single  exp_width=8  frac_width=24  explicit_period=on  period=1  equ=P=C  opselect=C  inp2=PCIN>>17  opr=+  inp1=P  carry=CIN  dbl_ovrd=off  block_type=constant
  Convert3 : xbsIndex_r4/Convert  gui_display_data_type=Fixed-point  arith_type="Signed  (2's comp)"  n_bits=16  bin_pt=14  float_type=Single  exp_bits=8  fraction_bits=24  quantization=Truncate  overflow=Wrap  en=off  latency=0  pipeline=on  dbl_ovrd=off  block_type=convert
  Convert4 : xbsIndex_r4/Convert  gui_display_data_type=Fixed-point  arith_type="Signed  (2's comp)"  n_bits=16  bin_pt=14  float_type=Single  exp_bits=8  fraction_bits=24  quantization=Truncate  overflow=Wrap  en=off  latency=0  pipeline=on  dbl_ovrd=off  block_type=convert
  Delay : xbsIndex_r4/Delay  rst=off  infoeditControl=Selection of Reset will increase slice count due to use of real FFs and instead of SRLs  en=off  latency=22  reg_retiming=off  dbl_ovrd=off  block_type=delay
  Delay1 : xbsIndex_r4/Delay  rst=off  infoeditControl=Selection of Reset will increase slice count due to use of real FFs and instead of SRLs  en=off  latency=1  reg_retiming=off  dbl_ovrd=off  block_type=delay
  Delay3 : xbsIndex_r4/Delay  rst=off  infoeditControl=Selection of Reset will increase slice count due to use of real FFs and instead of SRLs  en=off  latency=1  reg_retiming=off  dbl_ovrd=off  block_type=delay
  Register2 : xbsIndex_r4/Register  init=0  rst=off  en=on  dbl_ovrd=off  block_type=register
  Register4 : xbsIndex_r4/Register  init=0  rst=off  en=on  dbl_ovrd=off  block_type=register
  R : Outport
  Phase_out : Outport  Port=2
  A' : Outport  Port=3
  C_match_out : Outport  Port=4
  wires:
  Ain/1 -> Delay/1
  Delay/1 -> CORDIC 6.0 3/2
  Convert4/1 -> Register2/1
  CORDIC 6.0 3/2 -> Convert4/1
  Register2/1 -> R/1, CORDIC 6.0 3/3
  CORDIC 6.0 3/3 -> Convert3/1
  Constant5/1 -> CORDIC 6.0 3/1, CORDIC 6.0 3/4
  Register4/1 -> A'/1
  Convert3/1 -> Register4/1
  Phase/1 -> Delay1/1, CORDIC 6.0 3/5
  Delay3/1 -> Register2/2, C_match_out/1, Register4/2
  C_match_in/1 -> Delay3/1
  Delay1/1 -> Phase_out/1

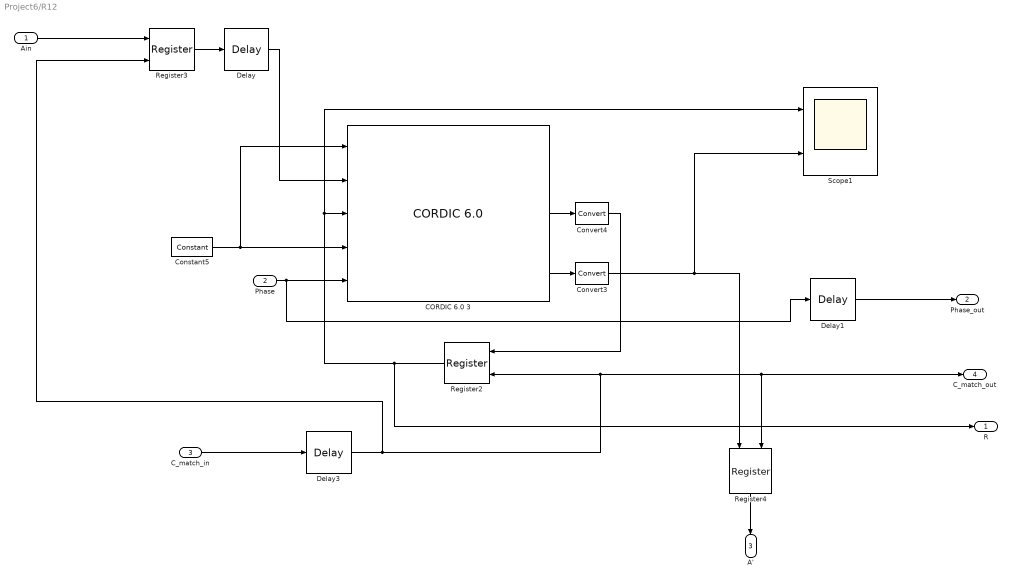
== system Project6/R12  ==
  Ain : Inport
  Phase : Inport  Port=2
  C_match_in : Inport  Port=3
  CORDIC 6.0 3 : xbsIndex_r4/CORDIC 6.0   functional_selection=Rotate  architectural_configuration=Parallel  pipelining_mode=Maximum  data_format=SignedFraction  phase_format=Radians  input_width=16  output_width=16  round_mode=Truncate  iterations=16  precision=16  compensation_scaling=LUT_based  coarse_rotation=on  aclken=off  aresetn=off  out_tready=off  cartesian_has_tuser=off  cartesian_has_tlast=off  cartesian_tuser_width=1  phase_has_tuser=off  phase_has_tlast=off  phase_tuser_width=1  out_tlast_behv=Null  flow_control=NonBlocking  optimize_goal=Performance  trim_axipin_name=on  ip_name=CORDIC  ip_version=6.0  dsptool_ready=true  ipcore_usecache=true  ipcore_useipmodelcache=true  wrapper_available=true  port_translation_map={ 'aclken' => 'en', 'aresetn' => 'rst' }  block_type=cordic_v6_0
      settings: infoedit=CORDIC 6.0
  Constant5 : xbsIndex_r4/Constant  const=1  gui_display_data_type=Boolean  arith_type=Boolean  n_bits=16  bin_pt=14  preci_type=Single  exp_width=8  frac_width=24  explicit_period=on  period=1  equ=P=C  opselect=C  inp2=PCIN>>17  opr=+  inp1=P  carry=CIN  dbl_ovrd=off  block_type=constant
  Convert3 : xbsIndex_r4/Convert  gui_display_data_type=Fixed-point  arith_type="Signed  (2's comp)"  n_bits=16  bin_pt=14  float_type=Single  exp_bits=8  fraction_bits=24  quantization=Truncate  overflow=Wrap  en=off  latency=0  pipeline=on  dbl_ovrd=off  block_type=convert
  Convert4 : xbsIndex_r4/Convert  gui_display_data_type=Fixed-point  arith_type="Signed  (2's comp)"  n_bits=16  bin_pt=14  float_type=Single  exp_bits=8  fraction_bits=24  quantization=Truncate  overflow=Wrap  en=off  latency=0  pipeline=on  dbl_ovrd=off  block_type=convert
  Delay : xbsIndex_r4/Delay  rst=off  infoeditControl=Selection of Reset will increase slice count due to use of real FFs and instead of SRLs  en=off  latency=22  reg_retiming=off  dbl_ovrd=off  block_type=delay
  Delay1 : xbsIndex_r4/Delay  rst=off  infoeditControl=Selection of Reset will increase slice count due to use of real FFs and instead of SRLs  en=off  latency=1  reg_retiming=off  dbl_ovrd=off  block_type=delay
  Delay3 : xbsIndex_r4/Delay  rst=off  infoeditControl=Selection of Reset will increase slice count due to use of real FFs and instead of SRLs  en=off  latency=1  reg_retiming=off  dbl_ovrd=off  block_type=delay
  Register2 : xbsIndex_r4/Register  init=0  rst=off  en=on  dbl_ovrd=off  block_type=register
  Register3 : xbsIndex_r4/Register  init=0  rst=off  en=on  dbl_ovrd=off  block_type=register
  Register4 : xbsIndex_r4/Register  init=0  rst=off  en=on  dbl_ovrd=off  block_type=register
  Scope1 : Scope  NumInputPorts=2
      settings: YMin=-5~-5  YMax=5~5  SaveName=ScopeData6
  R : Outport
  Phase_out : Outport  Port=2
  A' : Outport  Port=3
  C_match_out : Outport  Port=4
  wires:
  Ain/1 -> Register3/1
  Convert4/1 -> Register2/1
  CORDIC 6.0 3/2 -> Convert4/1
  CORDIC 6.0 3/3 -> Convert3/1
  Constant5/1 -> CORDIC 6.0 3/1, CORDIC 6.0 3/4
  Convert3/1 -> Scope1/2, Register4/1
  Phase/1 -> Delay1/1, CORDIC 6.0 3/5
  Delay3/1 -> Register3/2, Register2/2, C_match_out/1, Register4/2
  C_match_in/1 -> Delay3/1
  Delay1/1 -> Phase_out/1
  Register2/1 -> R/1, Scope1/1, CORDIC 6.0 3/3
  Delay/1 -> CORDIC 6.0 3/2
  Register3/1 -> Delay/1
  Register4/1 -> A'/1

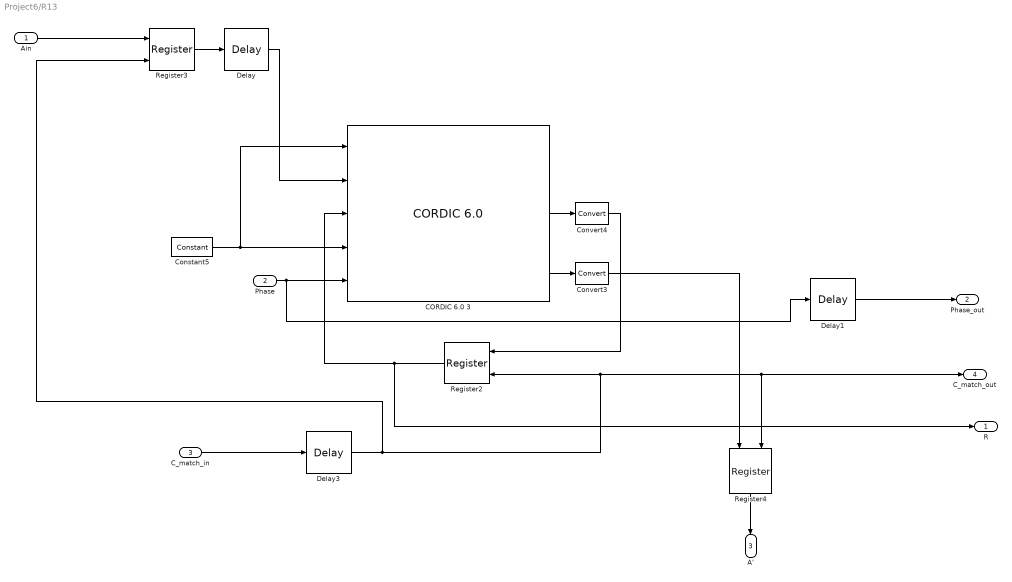
== system Project6/R13 ==
  Ain : Inport
  Phase : Inport  Port=2
  C_match_in : Inport  Port=3
  CORDIC 6.0 3 : xbsIndex_r4/CORDIC 6.0   functional_selection=Rotate  architectural_configuration=Parallel  pipelining_mode=Maximum  data_format=SignedFraction  phase_format=Radians  input_width=16  output_width=16  round_mode=Truncate  iterations=16  precision=16  compensation_scaling=LUT_based  coarse_rotation=on  aclken=off  aresetn=off  out_tready=off  cartesian_has_tuser=off  cartesian_has_tlast=off  cartesian_tuser_width=1  phase_has_tuser=off  phase_has_tlast=off  phase_tuser_width=1  out_tlast_behv=Null  flow_control=NonBlocking  optimize_goal=Performance  trim_axipin_name=on  ip_name=CORDIC  ip_version=6.0  dsptool_ready=true  ipcore_usecache=true  ipcore_useipmodelcache=true  wrapper_available=true  port_translation_map={ 'aclken' => 'en', 'aresetn' => 'rst' }  block_type=cordic_v6_0
      settings: infoedit=CORDIC 6.0
  Constant5 : xbsIndex_r4/Constant  const=1  gui_display_data_type=Boolean  arith_type=Boolean  n_bits=16  bin_pt=14  preci_type=Single  exp_width=8  frac_width=24  explicit_period=on  period=1  equ=P=C  opselect=C  inp2=PCIN>>17  opr=+  inp1=P  carry=CIN  dbl_ovrd=off  block_type=constant
  Convert3 : xbsIndex_r4/Convert  gui_display_data_type=Fixed-point  arith_type="Signed  (2's comp)"  n_bits=16  bin_pt=14  float_type=Single  exp_bits=8  fraction_bits=24  quantization=Truncate  overflow=Wrap  en=off  latency=0  pipeline=on  dbl_ovrd=off  block_type=convert
  Convert4 : xbsIndex_r4/Convert  gui_display_data_type=Fixed-point  arith_type="Signed  (2's comp)"  n_bits=16  bin_pt=14  float_type=Single  exp_bits=8  fraction_bits=24  quantization=Truncate  overflow=Wrap  en=off  latency=0  pipeline=on  dbl_ovrd=off  block_type=convert
  Delay : xbsIndex_r4/Delay  rst=off  infoeditControl=Selection of Reset will increase slice count due to use of real FFs and instead of SRLs  en=off  latency=22  reg_retiming=off  dbl_ovrd=off  block_type=delay
  Delay1 : xbsIndex_r4/Delay  rst=off  infoeditControl=Selection of Reset will increase slice count due to use of real FFs and instead of SRLs  en=off  latency=1  reg_retiming=off  dbl_ovrd=off  block_type=delay
  Delay3 : xbsIndex_r4/Delay  rst=off  infoeditControl=Selection of Reset will increase slice count due to use of real FFs and instead of SRLs  en=off  latency=1  reg_retiming=off  dbl_ovrd=off  block_type=delay
  Register2 : xbsIndex_r4/Register  init=0  rst=off  en=on  dbl_ovrd=off  block_type=register
  Register3 : xbsIndex_r4/Register  init=0  rst=off  en=on  dbl_ovrd=off  block_type=register
  Register4 : xbsIndex_r4/Register  init=0  rst=off  en=on  dbl_ovrd=off  block_type=register
  R : Outport
  Phase_out : Outport  Port=2
  A' : Outport  Port=3
  C_match_out : Outport  Port=4
  wires:
  Register3/1 -> Delay/1
  Ain/1 -> Register3/1
  Delay/1 -> CORDIC 6.0 3/2
  Convert4/1 -> Register2/1
  CORDIC 6.0 3/2 -> Convert4/1
  CORDIC 6.0 3/3 -> Convert3/1
  Constant5/1 -> CORDIC 6.0 3/1, CORDIC 6.0 3/4
  Register4/1 -> A'/1
  Convert3/1 -> Register4/1
  Phase/1 -> Delay1/1, CORDIC 6.0 3/5
  Delay3/1 -> Register3/2, Register2/2, C_match_out/1, Register4/2
  C_match_in/1 -> Delay3/1
  Delay1/1 -> Phase_out/1
  Register2/1 -> R/1, CORDIC 6.0 3/3

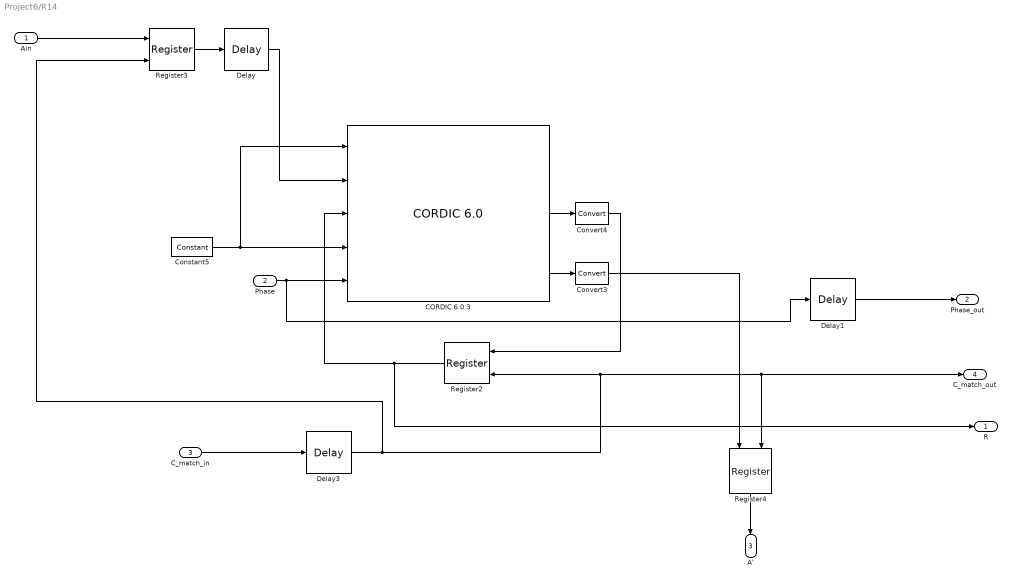
== system Project6/R14 ==
  Ain : Inport
  Phase : Inport  Port=2
  C_match_in : Inport  Port=3
  CORDIC 6.0 3 : xbsIndex_r4/CORDIC 6.0   functional_selection=Rotate  architectural_configuration=Parallel  pipelining_mode=Maximum  data_format=SignedFraction  phase_format=Radians  input_width=16  output_width=16  round_mode=Truncate  iterations=16  precision=16  compensation_scaling=LUT_based  coarse_rotation=on  aclken=off  aresetn=off  out_tready=off  cartesian_has_tuser=off  cartesian_has_tlast=off  cartesian_tuser_width=1  phase_has_tuser=off  phase_has_tlast=off  phase_tuser_width=1  out_tlast_behv=Null  flow_control=NonBlocking  optimize_goal=Performance  trim_axipin_name=on  ip_name=CORDIC  ip_version=6.0  dsptool_ready=true  ipcore_usecache=true  ipcore_useipmodelcache=true  wrapper_available=true  port_translation_map={ 'aclken' => 'en', 'aresetn' => 'rst' }  block_type=cordic_v6_0
      settings: infoedit=CORDIC 6.0
  Constant5 : xbsIndex_r4/Constant  const=1  gui_display_data_type=Boolean  arith_type=Boolean  n_bits=16  bin_pt=14  preci_type=Single  exp_width=8  frac_width=24  explicit_period=on  period=1  equ=P=C  opselect=C  inp2=PCIN>>17  opr=+  inp1=P  carry=CIN  dbl_ovrd=off  block_type=constant
  Convert3 : xbsIndex_r4/Convert  gui_display_data_type=Fixed-point  arith_type="Signed  (2's comp)"  n_bits=16  bin_pt=14  float_type=Single  exp_bits=8  fraction_bits=24  quantization=Truncate  overflow=Wrap  en=off  latency=0  pipeline=on  dbl_ovrd=off  block_type=convert
  Convert4 : xbsIndex_r4/Convert  gui_display_data_type=Fixed-point  arith_type="Signed  (2's comp)"  n_bits=16  bin_pt=14  float_type=Single  exp_bits=8  fraction_bits=24  quantization=Truncate  overflow=Wrap  en=off  latency=0  pipeline=on  dbl_ovrd=off  block_type=convert
  Delay : xbsIndex_r4/Delay  rst=off  infoeditControl=Selection of Reset will increase slice count due to use of real FFs and instead of SRLs  en=off  latency=22  reg_retiming=off  dbl_ovrd=off  block_type=delay
  Delay1 : xbsIndex_r4/Delay  rst=off  infoeditControl=Selection of Reset will increase slice count due to use of real FFs and instead of SRLs  en=off  latency=1  reg_retiming=off  dbl_ovrd=off  block_type=delay
  Delay3 : xbsIndex_r4/Delay  rst=off  infoeditControl=Selection of Reset will increase slice count due to use of real FFs and instead of SRLs  en=off  latency=1  reg_retiming=off  dbl_ovrd=off  block_type=delay
  Register2 : xbsIndex_r4/Register  init=0  rst=off  en=on  dbl_ovrd=off  block_type=register
  Register3 : xbsIndex_r4/Register  init=0  rst=off  en=on  dbl_ovrd=off  block_type=register
  Register4 : xbsIndex_r4/Register  init=0  rst=off  en=on  dbl_ovrd=off  block_type=register
  R : Outport
  Phase_out : Outport  Port=2
  A' : Outport  Port=3
  C_match_out : Outport  Port=4
  wires:
  Register3/1 -> Delay/1
  Ain/1 -> Register3/1
  Delay/1 -> CORDIC 6.0 3/2
  Convert4/1 -> Register2/1
  CORDIC 6.0 3/2 -> Convert4/1
  Register2/1 -> R/1, CORDIC 6.0 3/3
  CORDIC 6.0 3/3 -> Convert3/1
  Constant5/1 -> CORDIC 6.0 3/1, CORDIC 6.0 3/4
  Register4/1 -> A'/1
  Convert3/1 -> Register4/1
  Phase/1 -> Delay1/1, CORDIC 6.0 3/5
  Delay3/1 -> Register3/2, Register2/2, C_match_out/1, Register4/2
  C_match_in/1 -> Delay3/1
  Delay1/1 -> Phase_out/1

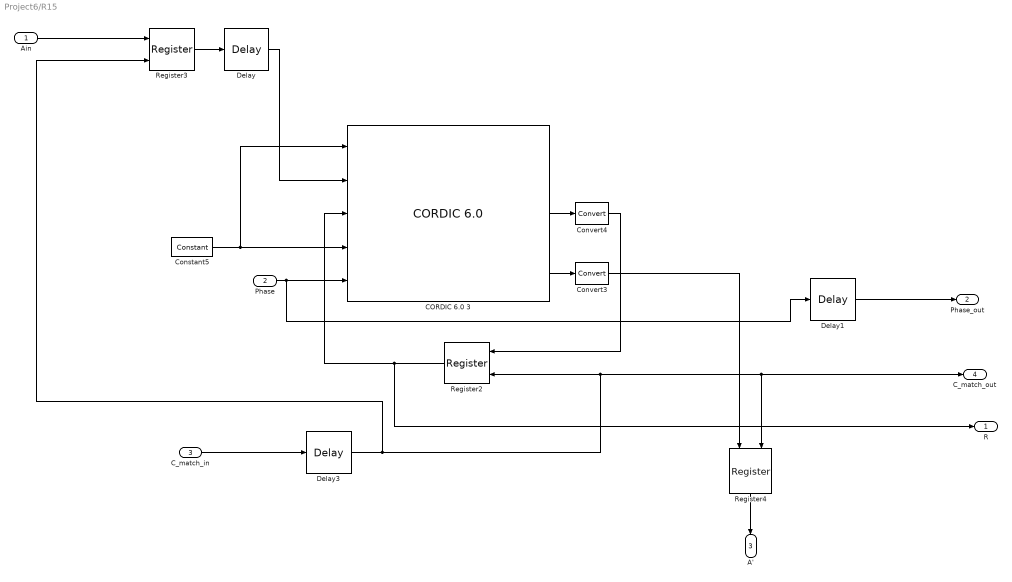
== system Project6/R15 ==
  Ain : Inport
  Phase : Inport  Port=2
  C_match_in : Inport  Port=3
  CORDIC 6.0 3 : xbsIndex_r4/CORDIC 6.0   functional_selection=Rotate  architectural_configuration=Parallel  pipelining_mode=Maximum  data_format=SignedFraction  phase_format=Radians  input_width=16  output_width=16  round_mode=Truncate  iterations=16  precision=16  compensation_scaling=LUT_based  coarse_rotation=on  aclken=off  aresetn=off  out_tready=off  cartesian_has_tuser=off  cartesian_has_tlast=off  cartesian_tuser_width=1  phase_has_tuser=off  phase_has_tlast=off  phase_tuser_width=1  out_tlast_behv=Null  flow_control=NonBlocking  optimize_goal=Performance  trim_axipin_name=on  ip_name=CORDIC  ip_version=6.0  dsptool_ready=true  ipcore_usecache=true  ipcore_useipmodelcache=true  wrapper_available=true  port_translation_map={ 'aclken' => 'en', 'aresetn' => 'rst' }  block_type=cordic_v6_0
      settings: infoedit=CORDIC 6.0
  Constant5 : xbsIndex_r4/Constant  const=1  gui_display_data_type=Boolean  arith_type=Boolean  n_bits=16  bin_pt=14  preci_type=Single  exp_width=8  frac_width=24  explicit_period=on  period=1  equ=P=C  opselect=C  inp2=PCIN>>17  opr=+  inp1=P  carry=CIN  dbl_ovrd=off  block_type=constant
  Convert3 : xbsIndex_r4/Convert  gui_display_data_type=Fixed-point  arith_type="Signed  (2's comp)"  n_bits=16  bin_pt=14  float_type=Single  exp_bits=8  fraction_bits=24  quantization=Truncate  overflow=Wrap  en=off  latency=0  pipeline=on  dbl_ovrd=off  block_type=convert
  Convert4 : xbsIndex_r4/Convert  gui_display_data_type=Fixed-point  arith_type="Signed  (2's comp)"  n_bits=16  bin_pt=14  float_type=Single  exp_bits=8  fraction_bits=24  quantization=Truncate  overflow=Wrap  en=off  latency=0  pipeline=on  dbl_ovrd=off  block_type=convert
  Delay : xbsIndex_r4/Delay  rst=off  infoeditControl=Selection of Reset will increase slice count due to use of real FFs and instead of SRLs  en=off  latency=22  reg_retiming=off  dbl_ovrd=off  block_type=delay
  Delay1 : xbsIndex_r4/Delay  rst=off  infoeditControl=Selection of Reset will increase slice count due to use of real FFs and instead of SRLs  en=off  latency=1  reg_retiming=off  dbl_ovrd=off  block_type=delay
  Delay3 : xbsIndex_r4/Delay  rst=off  infoeditControl=Selection of Reset will increase slice count due to use of real FFs and instead of SRLs  en=off  latency=1  reg_retiming=off  dbl_ovrd=off  block_type=delay
  Register2 : xbsIndex_r4/Register  init=0  rst=off  en=on  dbl_ovrd=off  block_type=register
  Register3 : xbsIndex_r4/Register  init=0  rst=off  en=on  dbl_ovrd=off  block_type=register
  Register4 : xbsIndex_r4/Register  init=0  rst=off  en=on  dbl_ovrd=off  block_type=register
  R : Outport
  Phase_out : Outport  Port=2
  A' : Outport  Port=3
  C_match_out : Outport  Port=4
  wires:
  Register3/1 -> Delay/1
  Ain/1 -> Register3/1
  Delay/1 -> CORDIC 6.0 3/2
  Convert4/1 -> Register2/1
  CORDIC 6.0 3/2 -> Convert4/1
  Register2/1 -> R/1, CORDIC 6.0 3/3
  CORDIC 6.0 3/3 -> Convert3/1
  Constant5/1 -> CORDIC 6.0 3/1, CORDIC 6.0 3/4
  Register4/1 -> A'/1
  Convert3/1 -> Register4/1
  Phase/1 -> Delay1/1, CORDIC 6.0 3/5
  Delay3/1 -> Register3/2, Register2/2, C_match_out/1, Register4/2
  C_match_in/1 -> Delay3/1
  Delay1/1 -> Phase_out/1
